simulink model "case_8_lead_car_stationary_ego_speedup25a"  (R2025b)
settings: Solver=VariableStepAuto  StartTime=0.0  StopTime=30  RelTol=1e-3
settings Model: Creator=jdcjd  LastModifiedBy=admin

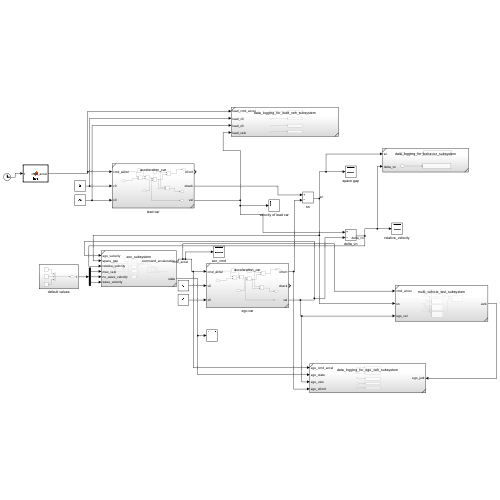
[thumbnail: Simulink's stored preview of the top-level diagram]
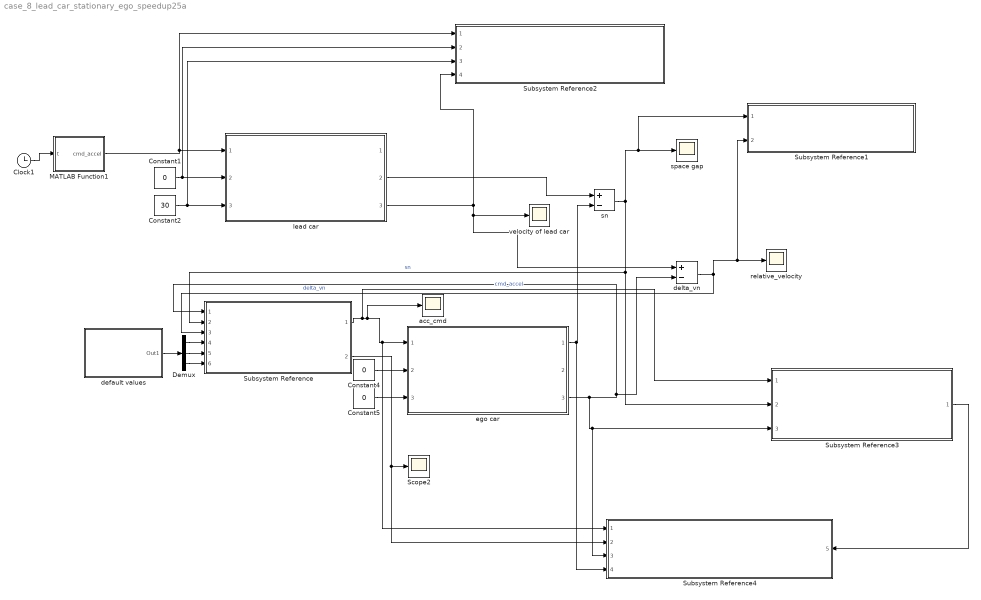
== system case_8_lead_car_stationary_ego_speedup25a ==
  Clock1 : Clock
  Constant1 : Constant  Value=0
  Constant2 : Constant  Value=30
  Constant4 : Constant  Value=0
  Constant5 : Constant  Value=0
  Demux : Demux  Outputs=3
  MATLAB Function1 : MATLAB Function  TreatAsAtomicUnit=on
  Scope2 : Scope
      settings: ActiveDisplayYMinimum=-1  ActiveDisplayYMaximum=1  DataLoggingVariableName=ScopeData2
  Subsystem Reference : Subsystem  ReferencedSubsystem=acc_subsystem
  Subsystem Reference1 : Subsystem  ReferencedSubsystem=data_logging_for_behavior_subsystem
  Subsystem Reference2 : Subsystem  ReferencedSubsystem=data_logging_for_lead_veh_subsystem
  Subsystem Reference3 : Subsystem  ReferencedSubsystem=multi_vehicle_test_subsystem
  Subsystem Reference4 : Subsystem  ReferencedSubsystem=data_logging_for_ego_veh_subsystem
      settings: PortSchema="{\"entries\":[{\"content\":{\"sides\":[{\"content\":{\"connectorIds\":[\"In1\",\"In2\",\"In3\",\"In4\"]},\"type\":\"ConnectorPlacement.EquallySpacedRectSide\",\"uuid\":\"1bb3a8cf-f981-4f8a-aff9-03896ccf7d7c\"},{\"content\":{\"connectorIds\":[\"In5\"],\"side\":\"RIGHT\"},\"type\":\"ConnectorPlacement.EquallySpacedRectSide\",\"uuid\":\"3f6ac5cb-96be-44a3-8993-3635a91bd658\"},{\"content\":{\"side\":\"TOP\"},\"type\":\"ConnectorPlacement.EquallySpacedRectSide\",\"uuid\":\"c641fc7f-a424-4033-b273-2526f6b205c0\"}]},\"type\":\"ConnectorPlacement.EquallySpacedConnector\",\"uuid\":\"2a4be48e-084e-4aa6-b74f-8fe234fedc1a\"}],\"packageUris\":[\"http://schema.mathworks.com/mf0/Connector/R2020b\"],\"version\":\"1.0\"}"
  acc_cmd : Scope
      settings: ActiveDisplayYMinimum=-3.1544938182907285  ActiveDisplayYMaximum=1.9958773488422277  DataLoggingVariableName=ScopeData3
  default values : Subsystem
  delta_vn : Sum  Inputs=+-
  ego car : Subsystem  ReferencedSubsystem=acceleration_car
  lead car : Subsystem  ReferencedSubsystem=acceleration_car
  relative_velocity : Scope
      settings: ActiveDisplayYMinimum=-6.7751153535477187  ActiveDisplayYMaximum=18.291496472530987
  sn : Sum  Inputs=+-
  space gap : Scope
      settings: ActiveDisplayYMinimum=-38.655422095716204  ActiveDisplayYMaximum=384.78877698816825
  velocity of lead car : Scope
      settings: ActiveDisplayYMinimum=-7.4781270427521109  ActiveDisplayYMaximum=67.303143384769015  DataLoggingVariableName=ScopeData4
  wires:
  Constant5/1 -> ego car/3
  Constant4/1 -> ego car/2
  ego car/3 -> Subsystem Reference4/3, Subsystem Reference3/3, Subsystem Reference/1, delta_vn/2
  Subsystem Reference/2 -> Subsystem Reference4/2, Scope2/1
  Subsystem Reference/1 -> Subsystem Reference3/1, acc_cmd/1, Subsystem Reference4/1, ego car/1  "cmd_accel"
  ego car/1 -> Subsystem Reference4/4, sn/2
  delta_vn/1 -> Subsystem Reference1/2, relative_velocity/1, Subsystem Reference/3  "delta_vn"
  MATLAB Function1/1(cmd_accel) -> Subsystem Reference2/1, lead car/1
  Constant1/1 -> Subsystem Reference2/2, lead car/2
  lead car/3 -> Subsystem Reference2/4, velocity of lead car/1, delta_vn/1
  sn/1 -> Subsystem Reference3/2, Subsystem Reference/2, Subsystem Reference1/1, space gap/1  "sn"
  Constant2/1 -> Subsystem Reference2/3, lead car/3
  Subsystem Reference3/1 -> Subsystem Reference4/5
  lead car/2 -> sn/1
  Clock1/1 -> MATLAB Function1/1(t)
  default values/1(Out1) -> Demux/1
  Demux/1 -> Subsystem Reference/4
  Demux/2 -> Subsystem Reference/5
  Demux/3 -> Subsystem Reference/6

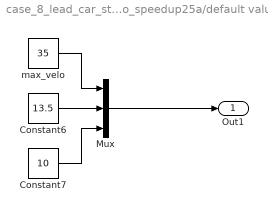
== system case_8_lead_car_stationary_ego_speedup25a/default values ==
  Constant6 : Constant  Value=13.5
  Constant7 : Constant  Value=10
  Mux : Mux  Inputs=3
  max_velo : Constant  Value=35
  Out1 : Outport
  wires:
  Constant7/1 -> Mux/3
  Constant6/1 -> Mux/2
  max_velo/1 -> Mux/1
  Mux/1 -> Out1/1

== matlab function case_8_lead_car_stationary_ego_speedup25a/MATLAB Function1 ==
  data: cmd_accel output; t input
function cmd_accel = fcn(t)
if t< 6
    cmd_accel = 0;
else
    cmd_accel = 2.5;
end
end
